simulink model "OUTPUT"  (R2025a)
settings: Solver=ode45  StartTime=0.0  StopTime=0.5  RelTol=1e-3  EnableMultiTasking=on
libraries: spsMosfetLib x7, spsSeriesRLCBranchLib x4, spsDCVoltageSourceLib x3, spsDiodeLib x3, spsVoltageMeasurementLib x1, sps_lib x1
settings Model: Creator=k c reddy  LastModifiedBy=gades
settings SolverCC: AlgebraicLoopSolver=TrustRegion
settings DataIOCC: LimitDataPoints=on  SaveFormat=Array  ReturnWorkspaceOutputs=off
settings OptimizationCC: LifeSpan=inf
settings DebuggingCC: UnconnectedInputMsg=warning  UnconnectedOutputMsg=warning  UnconnectedLineMsg=warning  SFUnexpectedBacktrackingDiag=warning  SFNoUnconditionalDefaultTransitionDiag=warning  SFExecutionAtInitializationDiag=none  ArithmeticOperatorsInVariantConditions=warning
settings HardwareCC: ProdBitPerPointer=32.0  ProdBitPerSizeT=32.0  ProdBitPerPtrDiffT=32.0  ProdLargestAtomicFloat=None  ProdIntDivRoundTo=Undefined  ProdEndianess=Unspecified  ProdWordSize=32.0  ProdHWDeviceType=32-bit Generic
settings ModelReferenceCC: PropagateSignalLabelsOutOfModel=off
settings SFSimCC: SimUseLocalCustomCode=off  CustomCodeUndefinedFunction=UseInterfaceOnly
settings RTWCC: RTWUseLocalCustomCode=off  GPUComputeCapability=3.5
settings CodeAppCC: StateflowObjectComments=on
settings GRTTargetCC: TargetLangStandard=C89/C90 (ANSI)
settings ConfigComp: CovMetricSettings=dw  CovSaveCumulativeToWorkspaceVar=on  CovSaveSingleToWorkspaceVar=on  CovExternalEMLEnable=off
settings SimscapeCC: SimscapeNormalizeSystem=off

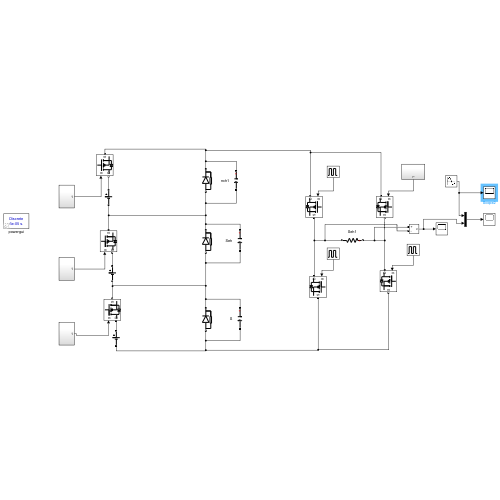
[thumbnail: Simulink's stored preview of the top-level diagram]
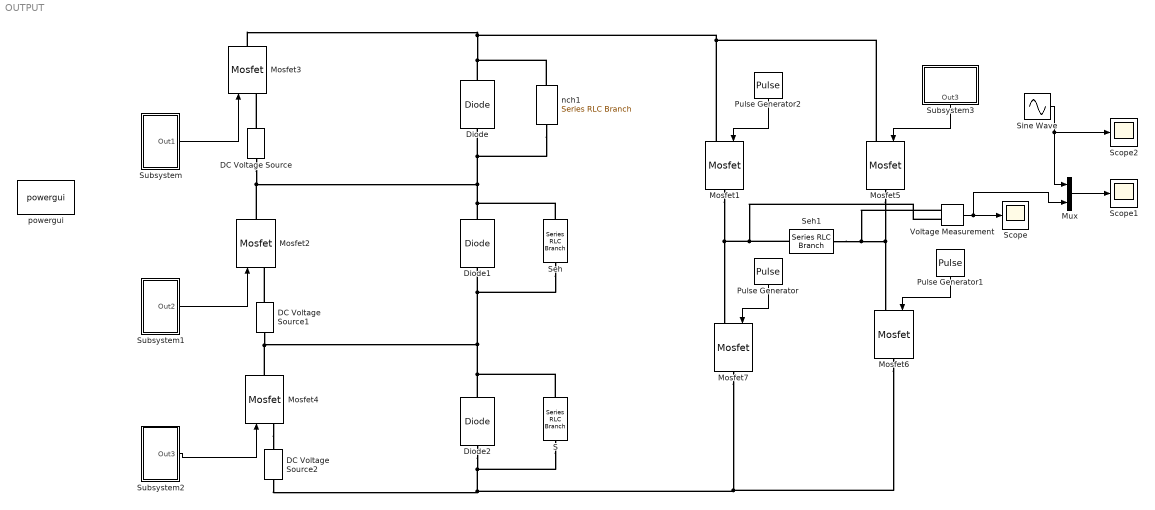
== system OUTPUT ==
  DC Voltage Source : spsDCVoltageSourceLib/DC Voltage Source  Amplitude=12  Measurements=None
  DC Voltage Source1 : spsDCVoltageSourceLib/DC Voltage Source  Amplitude=24  Measurements=None
  DC Voltage Source2 : spsDCVoltageSourceLib/DC Voltage Source  Amplitude=48  Measurements=None
  Diode : spsDiodeLib/Diode  Ron=0.001  Lon=0  Vf=0.8  IC=0  UseSnubber=off  Rs=500  Cs=250e-9  Measurements=off
  Diode1 : spsDiodeLib/Diode  Ron=0.001  Lon=0  Vf=0.8  IC=0  UseSnubber=off  Rs=500  Cs=250e-9  Measurements=off
  Diode2 : spsDiodeLib/Diode  Ron=0.001  Lon=0  Vf=0.8  IC=0  UseSnubber=off  Rs=500  Cs=250e-9  Measurements=off
  Mosfet{1..7} (7 alike) : spsMosfetLib/Mosfet  Ron=0.1  Lon=0  Rd=0.01  Vfd=0  IC=0  Rs=1e5  Cs=inf  Measurements=off
  Mux : Mux  Inputs=2
  Pulse Generator : DiscretePulseGenerator  PulseType=Time based  Period=20e-3  PulseWidth=13/28*100  PhaseDelay=15/28*20e-3
  Pulse Generator1 : DiscretePulseGenerator  PulseType=Time based  Period=20e-3  PulseWidth=13/28*100  PhaseDelay=1/28*20e-3
  Pulse Generator2 : DiscretePulseGenerator  PulseType=Time based  Period=20e-3  PulseWidth=15/28*100
  S : spsSeriesRLCBranchLib/Series RLC Branch  LConnTagsString=__new0  RConnTagsString=__new0  BranchType=C  Resistance=1  Inductance=1e-3  SetiL0=off  InitialCurrent=0  Capacitance=100e-9  Setx0=off  InitialVoltage=0  Measurements=None
  Scope : Scope
      settings: TimeSpan=0.04711701149425285  ActiveDisplayYMinimum=-257.1555459782511  ActiveDisplayYMaximum=142.96001861956961  DataLoggingSaveFormat=Array
  Scope1 : Scope
      settings: TimeSpan=0.04711701149425285  ActiveDisplayYMinimum=-228.5738506759055  ActiveDisplayYMaximum=246.62048252639613  DataLoggingSaveFormat=Array
  Scope2 : Scope
      settings: TimeSpan=0.04711701149425285  ActiveDisplayYMinimum=-356.517052102668  ActiveDisplayYMaximum=711.58282210294715  DataLoggingVariableName=ScopeData2  DataLoggingSaveFormat=Array
  Seh : spsSeriesRLCBranchLib/Series RLC Branch  LConnTagsString=__new0  RConnTagsString=__new0  BranchType=C  Resistance=1  Inductance=1e-3  SetiL0=off  InitialCurrent=0  Capacitance=100e-9  Setx0=off  InitialVoltage=0  Measurements=None
  Seh1 : spsSeriesRLCBranchLib/Series RLC Branch  LConnTagsString=__new0  RConnTagsString=__new0  BranchType=R  Resistance=100  Inductance=1e-3  SetiL0=off  InitialCurrent=0  Capacitance=1e-6  Setx0=off  InitialVoltage=0  Measurements=None
  Sine Wave : Sin  Amplitude=80  Frequency=50*2*pi  Phase=(120/360)*100  SampleTime=0
  Subsystem : Subsystem
  Subsystem1 : Subsystem
  Subsystem2 : Subsystem
  Subsystem3 : Subsystem
  Voltage Measurement : spsVoltageMeasurementLib/Voltage Measurement  PhasorSimulation=off  OutputType=Complex  PSBequivalent=0
  nch1 : spsSeriesRLCBranchLib/Series RLC Branch  LConnTagsString=__new0  RConnTagsString=__new0  BranchType=C  Resistance=1  Inductance=1e-3  SetiL0=off  InitialCurrent=0  Capacitance=100e-9  Setx0=off  InitialVoltage=0  Measurements=None
  powergui : sps_lib/powergui  Priority=1  SimulationMode=Discrete  SampleTime=50e-6  frequency=60  Iterations=50  frequencyindice=0  Pbase=100e6  ErrMax=1e-4  UnitsV=kV  UnitsW=MW  buscounter=0  FunctionMessages=off  echomessages=off  EnableUseOfTLC=off  CurrentSourceSwitches=off  DisableSnubberDevices=off  DisableRonSwitches=off  DisableVfSwitches=off  DisplayEquations=off  AutomaticDiscreteSolvers=off  SolverType=Tustin/Backward Euler (TBE)  Interpol=off  ExternalGateDelay=off  methode=off  Ts=100  x0status=blocks  SPID=off  SwTol=0  HookPort=off  NonlinearTolerance=1e-4  nMaxIteration=100  ContinueOnMaxIteration=off  RestoreLinks=warning  ResistiveCurrentMeasurement=off  Frange=[0:2:500]  Ylog=off  Xlog=on  ShowGrid=off  save=off  variable=ZData  structure=0  ZoomFFT=off  StartTime=0.0  cycles=1  DisplayStyle=1  fundamental=60  FreqAxis=off  MaxFrequency=1000  frequencyindicesteady=1  RmsSteady=1  display=off
  wires:
  Subsystem/1(Out1) -> Mosfet3/1
  Subsystem1/1(Out2) -> Mosfet2/1
  Subsystem2/1(Out3) -> Mosfet4/1
  Pulse Generator/1 -> Mosfet7/1
  Pulse Generator1/1 -> Mosfet6/1
  Pulse Generator2/1 -> Mosfet1/1
  Subsystem3/1(Out3) -> Mosfet5/1
  Voltage Measurement/1 -> Mux/2, Scope/1
  Sine Wave/1 -> Mux/1, Scope2/1
  Mux/1 -> Scope1/1
  connections:
  DC Voltage Source/RConn1 -- Mosfet3/LConn1
  DC Voltage Source1/RConn1 -- Mosfet2/LConn1
  Mosfet4/LConn1 -- DC Voltage Source2/RConn1
  Diode2/RConn1 -- Mosfet4/RConn1 -- DC Voltage Source1/LConn1 -- Seh/RConn1 -- Diode1/LConn1 -- S/LConn1
  Diode1/RConn1 -- Mosfet2/RConn1 -- DC Voltage Source/LConn1 -- nch1/RConn1 -- Diode/LConn1 -- Seh/LConn1
  Diode2/LConn1 -- Mosfet6/RConn1 -- Mosfet7/RConn1 -- DC Voltage Source2/LConn1 -- S/RConn1
  nch1/LConn1 -- Mosfet5/LConn1 -- Mosfet1/LConn1 -- Mosfet3/RConn1 -- Diode/RConn1
  Mosfet5/RConn1 -- Voltage Measurement/LConn1 -- Seh1/LConn1 -- Mosfet6/LConn1
  Mosfet1/RConn1 -- Voltage Measurement/LConn2 -- Seh1/RConn1 -- Mosfet7/LConn1

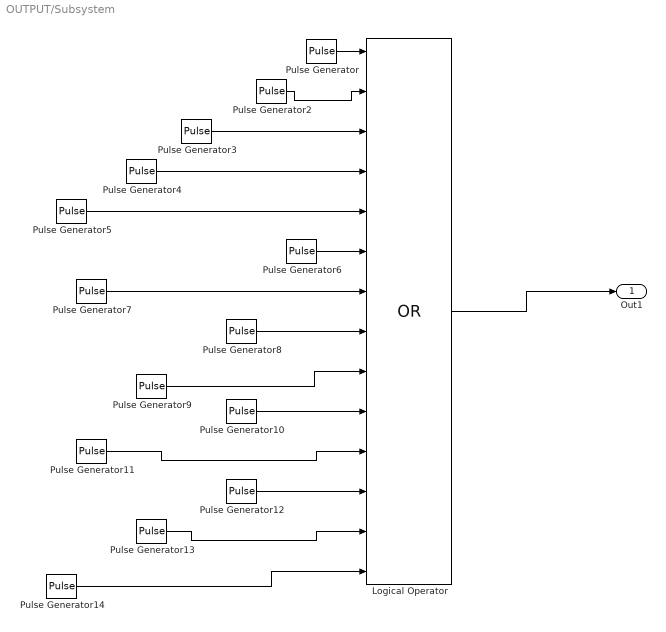
== system OUTPUT/Subsystem ==
  Logical Operator : Logic  Operator=OR  Inputs=14  AllPortsSameDT=off  OutDataTypeStr=boolean
  Pulse Generator : DiscretePulseGenerator  PulseType=Time based  Period=20e-3  PulseWidth=3.5714  PhaseDelay=0.7143e-3
  Pulse Generator10 : DiscretePulseGenerator  PulseType=Time based  Period=20e-3  PulseWidth=3.5714  PhaseDelay=19/28*20e-3
  Pulse Generator11 : DiscretePulseGenerator  PulseType=Time based  Period=20e-3  PulseWidth=3.5714  PhaseDelay=21/28*20e-3
  Pulse Generator12 : DiscretePulseGenerator  PulseType=Time based  Period=20e-3  PulseWidth=3.5714  PhaseDelay=23/28*20e-3
  Pulse Generator13 : DiscretePulseGenerator  PulseType=Time based  Period=20e-3  PulseWidth=3.5714  PhaseDelay=25/28*20e-3
  Pulse Generator14 : DiscretePulseGenerator  PulseType=Time based  Period=20e-3  PulseWidth=3.5714  PhaseDelay=27/28*20e-3
  Pulse Generator2 : DiscretePulseGenerator  PulseType=Time based  Period=20e-3  PulseWidth=3.5714  PhaseDelay=3/28*20e-3
  Pulse Generator3 : DiscretePulseGenerator  PulseType=Time based  Period=20e-3  PulseWidth=3.5714  PhaseDelay=5/28*20e-3
  Pulse Generator4 : DiscretePulseGenerator  PulseType=Time based  Period=20e-3  PulseWidth=3.5714  PhaseDelay=7/28*20e-3
  Pulse Generator5 : DiscretePulseGenerator  PulseType=Time based  Period=20e-3  PulseWidth=3.5714  PhaseDelay=9/28*20e-3
  Pulse Generator6 : DiscretePulseGenerator  PulseType=Time based  Period=20e-3  PulseWidth=3.5714  PhaseDelay=11/28*20e-3
  Pulse Generator7 : DiscretePulseGenerator  PulseType=Time based  Period=20e-3  PulseWidth=3.5714  PhaseDelay=13/28*20e-3
  Pulse Generator8 : DiscretePulseGenerator  PulseType=Time based  Period=20e-3  PulseWidth=3.5714  PhaseDelay=15/28*20e-3
  Pulse Generator9 : DiscretePulseGenerator  PulseType=Time based  Period=20e-3  PulseWidth=3.5714  PhaseDelay=17/28*20e-3
  Out1 : Outport
  wires:
  Pulse Generator10/1 -> Logical Operator/10
  Pulse Generator9/1 -> Logical Operator/9
  Pulse Generator13/1 -> Logical Operator/13
  Pulse Generator8/1 -> Logical Operator/8
  Pulse Generator11/1 -> Logical Operator/11
  Pulse Generator14/1 -> Logical Operator/14
  Logical Operator/1 -> Out1/1
  Pulse Generator6/1 -> Logical Operator/6
  Pulse Generator3/1 -> Logical Operator/3
  Pulse Generator5/1 -> Logical Operator/5
  Pulse Generator4/1 -> Logical Operator/4
  Pulse Generator7/1 -> Logical Operator/7
  Pulse Generator/1 -> Logical Operator/1
  Pulse Generator2/1 -> Logical Operator/2
  Pulse Generator12/1 -> Logical Operator/12

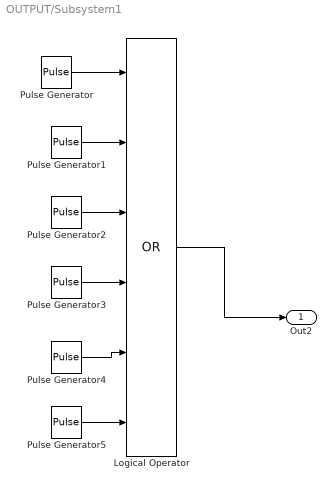
== system OUTPUT/Subsystem1 ==
  Logical Operator : Logic  Operator=OR  Inputs=6  AllPortsSameDT=off  OutDataTypeStr=boolean
  Pulse Generator : DiscretePulseGenerator  PulseType=Time based  Period=20e-3  PulseWidth=2/28*100  PhaseDelay=2/28*20e-3
  Pulse Generator1 : DiscretePulseGenerator  PulseType=Time based  Period=20e-3  PulseWidth=3/28*100  PhaseDelay=6/28*20e-3
  Pulse Generator2 : DiscretePulseGenerator  PulseType=Time based  Period=20e-3  PulseWidth=2/28*100  PhaseDelay=11/28*20e-3
  Pulse Generator3 : DiscretePulseGenerator  PulseType=Time based  Period=20e-3  PulseWidth=2/28*100  PhaseDelay=16/28*20e-3
  Pulse Generator4 : DiscretePulseGenerator  PulseType=Time based  Period=20e-3  PulseWidth=3/28*100  PhaseDelay=20/28*20e-3
  Pulse Generator5 : DiscretePulseGenerator  PulseType=Time based  Period=20e-3  PulseWidth=2/28*100  PhaseDelay=25/28*20e-3
  Out2 : Outport
  wires:
  Logical Operator/1 -> Out2/1
  Pulse Generator4/1 -> Logical Operator/5
  Pulse Generator/1 -> Logical Operator/1
  Pulse Generator2/1 -> Logical Operator/3
  Pulse Generator1/1 -> Logical Operator/2
  Pulse Generator3/1 -> Logical Operator/4
  Pulse Generator5/1 -> Logical Operator/6

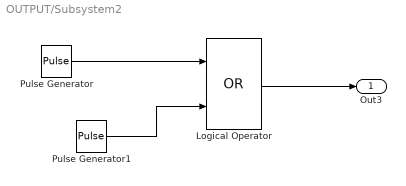
== system OUTPUT/Subsystem2 ==
  Logical Operator : Logic  Operator=OR  AllPortsSameDT=off  OutDataTypeStr=boolean
  Pulse Generator : DiscretePulseGenerator  PulseType=Time based  Period=20e-3  PulseWidth=7/28*100  PhaseDelay=4/28*20e-3
  Pulse Generator1 : DiscretePulseGenerator  PulseType=Time based  Period=20e-3  PulseWidth=7/28*100  PhaseDelay=18/28*20e-3
  Out3 : Outport
  wires:
  Logical Operator/1 -> Out3/1
  Pulse Generator1/1 -> Logical Operator/2
  Pulse Generator/1 -> Logical Operator/1

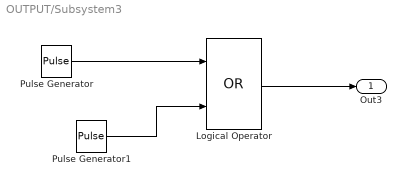
== system OUTPUT/Subsystem3 ==
  Logical Operator : Logic  Operator=OR  AllPortsSameDT=off  OutDataTypeStr=boolean
  Pulse Generator : DiscretePulseGenerator  PulseType=Time based  Period=20e-3  PulseWidth=1/28*100
  Pulse Generator1 : DiscretePulseGenerator  PulseType=Time based  Period=20e-3  PulseWidth=14/28*100  PhaseDelay=15/28*20e-3
  Out3 : Outport
  wires:
  Pulse Generator/1 -> Logical Operator/1
  Pulse Generator1/1 -> Logical Operator/2
  Logical Operator/1 -> Out3/1
